simulink model "stepResponse"  (R2021a)
settings: configuration reference "ctrlConfigSet" (kept outside this file)
settings Model: DataDictionary=stepResponseData.sldd  Creator=The MathWorks, Inc.  LastModifiedBy=hgu8
settings ConfigSetRef: SourceName=ctrlConfigSet

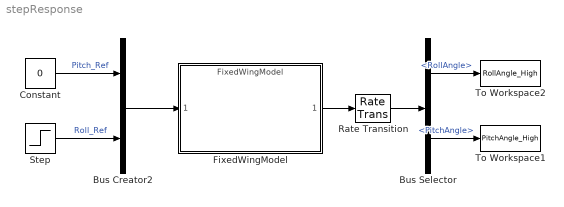
== system stepResponse ==
  Bus Creator2 : BusCreator  Inputs=2  OutDataTypeStr=Bus: FixedWingControlBus2  NonVirtualBus=on
  Bus Selector : BusSelector  OutputSignals=RollAngle,PitchAngle
  Constant : Constant  Value=0
  FixedWingModel : ModelReference  ModelNameDialog=FixedWingModel  SimulationMode=Normal  ModelReferenceVersion=3.52
  Rate Transition : RateTransition  OutPortSampleTime=0.1
  Step : Step  After=9.3  SampleTime=0
  To Workspace1 : ToWorkspace  VariableName=PitchAngle_High  SaveFormat=Timeseries  SampleTime=-1
  To Workspace2 : ToWorkspace  VariableName=RollAngle_High  SaveFormat=Timeseries  SampleTime=-1
  wires:
  Bus Selector/2 -> To Workspace1/1  "<PitchAngle>"
  Bus Selector/1 -> To Workspace2/1  "<RollAngle>"
  FixedWingModel/1 -> Rate Transition/1
  Rate Transition/1 -> Bus Selector/1
  Bus Creator2/1 -> FixedWingModel/1
  Step/1 -> Bus Creator2/2  "Roll_Ref"
  Constant/1 -> Bus Creator2/1  "Pitch_Ref"
